simulink model "traffic_light"  (R2020a)
settings: Solver=VariableStepAuto  StartTime=0.0  StopTime=150  RelTol=1e-3
settings Model: Creator=naina  LastModifiedBy=naina

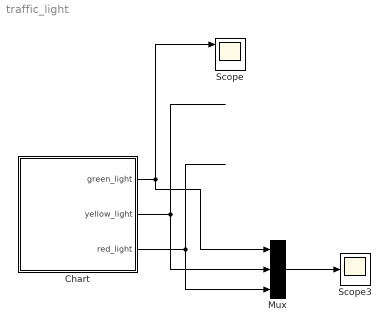
== system traffic_light ==
  Chart : Stateflow chart  TreatAsAtomicUnit=on
  Mux : Mux  Inputs=3
  Scope : Scope  NumInputPorts=3
  Scope3 : Scope
  wires:
  Chart/1(green_light) -> Scope/1, Mux/1
  Chart/2(yellow_light) -> Mux/2
  Chart/3(red_light) -> Mux/3
  Mux/1 -> Scope3/1

== stateflow chart traffic_light/Chart ==
  state YELLOW
    entry:
    red_light=0;
    green_light=0;
    yellow_light=1;
  state RED
    entry:
    red_light=1;
    green_light=0;
    yellow_light=0;
  state GREEN
    entry:
    red_light=0;
    green_light=1;
    yellow_light=0;
  (default) -> RED
  YELLOW -> RED : after(3,sec)
  GREEN -> YELLOW : after(50,sec)
  RED -> GREEN : after(50,sec)
  data: green_light output; yellow_light output; red_light output
